simulink model "rx2"  (R2022b)
settings: Solver=FixedStepDiscrete  StartTime=0.0  StopTime=3.3E6  FixedStep=1  RelTol=1e-3  EnableMultiTasking=on
model workspace (MAT data in the model file):
  mwTaskManagerKernelLatency = 0
undefined symbols (not defined in the file or in its folder): Add, jsin, magnitude, rom_pilot_conj_tt, Shift
libraries: hdlsllib x3231, whdlutilities x525, simulink x260, whdlmod x112, whdledac x26, dsphdlmathfun2 x24, commchan3 x1
(part 18 of 59)

== system rx2/process divide/transport_block5/Subsystem1/ctrl_gen ==
  data_in : Inport
  valid_in : Inport  Port=2
  Delay : Delay  DelayLength=1  InitialCondition=0
  Delay1 : Delay  DelayLength=1  InitialCondition=0
  Delay2 : Delay  DelayLength=1  InitialCondition=0
  Detect Fall Nonpositive : hdlsllib/Logic and Bit Operations/Detect Fall Nonpositive  vinit=0  OutDataTypeStr=boolean
  Detect Rise Positive : hdlsllib/Logic and Bit Operations/Detect Rise Positive  vinit=0  OutDataTypeStr=boolean
  Sample Control Bus Creator : whdlutilities/Sample Control Bus Creator
  data_out : Outport
  ctrl_out : Outport  Port=2
  wires:
  Detect Fall Nonpositive/1 -> Sample Control Bus Creator/2
  valid_in/1 -> Delay/1, Detect Fall Nonpositive/1, Delay1/1
  Sample Control Bus Creator/1 -> ctrl_out/1
  Delay/1 -> Sample Control Bus Creator/3
  Delay1/1 -> Detect Rise Positive/1
  data_in/1 -> Delay2/1
  Delay2/1 -> data_out/1
  Detect Rise Positive/1 -> Sample Control Bus Creator/1

== system rx2/process divide/transport_block5/Subsystem10/ctrl_gen ==
  data_in : Inport
  valid_in : Inport  Port=2
  Delay : Delay  DelayLength=1  InitialCondition=0
  Delay1 : Delay  DelayLength=1  InitialCondition=0
  Delay2 : Delay  DelayLength=1  InitialCondition=0
  Detect Fall Nonpositive : hdlsllib/Logic and Bit Operations/Detect Fall Nonpositive  vinit=0  OutDataTypeStr=boolean
  Detect Rise Positive : hdlsllib/Logic and Bit Operations/Detect Rise Positive  vinit=0  OutDataTypeStr=boolean
  Sample Control Bus Creator : whdlutilities/Sample Control Bus Creator
  data_out : Outport
  ctrl_out : Outport  Port=2
  wires:
  Detect Rise Positive/1 -> Sample Control Bus Creator/1
  Delay2/1 -> data_out/1
  data_in/1 -> Delay2/1
  Delay1/1 -> Detect Rise Positive/1
  Delay/1 -> Sample Control Bus Creator/3
  Sample Control Bus Creator/1 -> ctrl_out/1
  valid_in/1 -> Delay1/1, Detect Fall Nonpositive/1, Delay/1
  Detect Fall Nonpositive/1 -> Sample Control Bus Creator/2

== system rx2/process divide/transport_block5/Subsystem11/ctrl_gen ==
  data_in : Inport
  valid_in : Inport  Port=2
  Delay : Delay  DelayLength=1  InitialCondition=0
  Delay1 : Delay  DelayLength=1  InitialCondition=0
  Delay2 : Delay  DelayLength=1  InitialCondition=0
  Detect Fall Nonpositive : hdlsllib/Logic and Bit Operations/Detect Fall Nonpositive  vinit=0  OutDataTypeStr=boolean
  Detect Rise Positive : hdlsllib/Logic and Bit Operations/Detect Rise Positive  vinit=0  OutDataTypeStr=boolean
  Sample Control Bus Creator : whdlutilities/Sample Control Bus Creator
  data_out : Outport
  ctrl_out : Outport  Port=2
  wires:
  Detect Rise Positive/1 -> Sample Control Bus Creator/1
  Delay2/1 -> data_out/1
  data_in/1 -> Delay2/1
  Delay1/1 -> Detect Rise Positive/1
  Delay/1 -> Sample Control Bus Creator/3
  Sample Control Bus Creator/1 -> ctrl_out/1
  valid_in/1 -> Delay1/1, Detect Fall Nonpositive/1, Delay/1
  Detect Fall Nonpositive/1 -> Sample Control Bus Creator/2

== system rx2/process divide/transport_block5/Subsystem12/ctrl_gen ==
  data_in : Inport
  valid_in : Inport  Port=2
  Delay : Delay  DelayLength=1  InitialCondition=0
  Delay1 : Delay  DelayLength=1  InitialCondition=0
  Delay2 : Delay  DelayLength=1  InitialCondition=0
  Detect Fall Nonpositive : hdlsllib/Logic and Bit Operations/Detect Fall Nonpositive  vinit=0  OutDataTypeStr=boolean
  Detect Rise Positive : hdlsllib/Logic and Bit Operations/Detect Rise Positive  vinit=0  OutDataTypeStr=boolean
  Sample Control Bus Creator : whdlutilities/Sample Control Bus Creator
  data_out : Outport
  ctrl_out : Outport  Port=2
  wires:
  Detect Rise Positive/1 -> Sample Control Bus Creator/1
  Delay2/1 -> data_out/1
  data_in/1 -> Delay2/1
  Delay1/1 -> Detect Rise Positive/1
  Delay/1 -> Sample Control Bus Creator/3
  Sample Control Bus Creator/1 -> ctrl_out/1
  valid_in/1 -> Delay1/1, Detect Fall Nonpositive/1, Delay/1
  Detect Fall Nonpositive/1 -> Sample Control Bus Creator/2

== system rx2/process divide/transport_block5/Subsystem13/ctrl_gen ==
  data_in : Inport
  valid_in : Inport  Port=2
  Delay : Delay  DelayLength=1  InitialCondition=0
  Delay1 : Delay  DelayLength=1  InitialCondition=0
  Delay2 : Delay  DelayLength=1  InitialCondition=0
  Detect Fall Nonpositive : hdlsllib/Logic and Bit Operations/Detect Fall Nonpositive  vinit=0  OutDataTypeStr=boolean
  Detect Rise Positive : hdlsllib/Logic and Bit Operations/Detect Rise Positive  vinit=0  OutDataTypeStr=boolean
  Sample Control Bus Creator : whdlutilities/Sample Control Bus Creator
  data_out : Outport
  ctrl_out : Outport  Port=2
  wires:
  Detect Rise Positive/1 -> Sample Control Bus Creator/1
  Delay2/1 -> data_out/1
  data_in/1 -> Delay2/1
  Delay1/1 -> Detect Rise Positive/1
  Delay/1 -> Sample Control Bus Creator/3
  Sample Control Bus Creator/1 -> ctrl_out/1
  valid_in/1 -> Delay1/1, Detect Fall Nonpositive/1, Delay/1
  Detect Fall Nonpositive/1 -> Sample Control Bus Creator/2

== system rx2/process divide/transport_block5/Subsystem14/ctrl_gen ==
  data_in : Inport
  valid_in : Inport  Port=2
  Delay : Delay  DelayLength=1  InitialCondition=0
  Delay1 : Delay  DelayLength=1  InitialCondition=0
  Delay2 : Delay  DelayLength=1  InitialCondition=0
  Detect Fall Nonpositive : hdlsllib/Logic and Bit Operations/Detect Fall Nonpositive  vinit=0  OutDataTypeStr=boolean
  Detect Rise Positive : hdlsllib/Logic and Bit Operations/Detect Rise Positive  vinit=0  OutDataTypeStr=boolean
  Sample Control Bus Creator : whdlutilities/Sample Control Bus Creator
  data_out : Outport
  ctrl_out : Outport  Port=2
  wires:
  Detect Rise Positive/1 -> Sample Control Bus Creator/1
  Delay2/1 -> data_out/1
  data_in/1 -> Delay2/1
  Delay1/1 -> Detect Rise Positive/1
  Delay/1 -> Sample Control Bus Creator/3
  Sample Control Bus Creator/1 -> ctrl_out/1
  valid_in/1 -> Delay1/1, Detect Fall Nonpositive/1, Delay/1
  Detect Fall Nonpositive/1 -> Sample Control Bus Creator/2

== system rx2/process divide/transport_block5/Subsystem2/ctrl_gen ==
  data_in : Inport
  valid_in : Inport  Port=2
  Delay : Delay  DelayLength=1  InitialCondition=0
  Delay1 : Delay  DelayLength=1  InitialCondition=0
  Delay2 : Delay  DelayLength=1  InitialCondition=0
  Detect Fall Nonpositive : hdlsllib/Logic and Bit Operations/Detect Fall Nonpositive  vinit=0  OutDataTypeStr=boolean
  Detect Rise Positive : hdlsllib/Logic and Bit Operations/Detect Rise Positive  vinit=0  OutDataTypeStr=boolean
  Sample Control Bus Creator : whdlutilities/Sample Control Bus Creator
  data_out : Outport
  ctrl_out : Outport  Port=2
  wires:
  Detect Rise Positive/1 -> Sample Control Bus Creator/1
  Delay2/1 -> data_out/1
  data_in/1 -> Delay2/1
  Delay1/1 -> Detect Rise Positive/1
  Delay/1 -> Sample Control Bus Creator/3
  Sample Control Bus Creator/1 -> ctrl_out/1
  valid_in/1 -> Delay1/1, Detect Fall Nonpositive/1, Delay/1
  Detect Fall Nonpositive/1 -> Sample Control Bus Creator/2

== system rx2/process divide/transport_block5/Subsystem3/ctrl_gen ==
  data_in : Inport
  valid_in : Inport  Port=2
  Delay : Delay  DelayLength=1  InitialCondition=0
  Delay1 : Delay  DelayLength=1  InitialCondition=0
  Delay2 : Delay  DelayLength=1  InitialCondition=0
  Detect Fall Nonpositive : hdlsllib/Logic and Bit Operations/Detect Fall Nonpositive  vinit=0  OutDataTypeStr=boolean
  Detect Rise Positive : hdlsllib/Logic and Bit Operations/Detect Rise Positive  vinit=0  OutDataTypeStr=boolean
  Sample Control Bus Creator : whdlutilities/Sample Control Bus Creator
  data_out : Outport
  ctrl_out : Outport  Port=2
  wires:
  Detect Fall Nonpositive/1 -> Sample Control Bus Creator/2
  valid_in/1 -> Delay/1, Detect Fall Nonpositive/1, Delay1/1
  Sample Control Bus Creator/1 -> ctrl_out/1
  Delay/1 -> Sample Control Bus Creator/3
  Delay1/1 -> Detect Rise Positive/1
  data_in/1 -> Delay2/1
  Delay2/1 -> data_out/1
  Detect Rise Positive/1 -> Sample Control Bus Creator/1

== system rx2/process divide/transport_block5/Subsystem4/ctrl_gen ==
  data_in : Inport
  valid_in : Inport  Port=2
  Delay : Delay  DelayLength=1  InitialCondition=0
  Delay1 : Delay  DelayLength=1  InitialCondition=0
  Delay2 : Delay  DelayLength=1  InitialCondition=0
  Detect Fall Nonpositive : hdlsllib/Logic and Bit Operations/Detect Fall Nonpositive  vinit=0  OutDataTypeStr=boolean
  Detect Rise Positive : hdlsllib/Logic and Bit Operations/Detect Rise Positive  vinit=0  OutDataTypeStr=boolean
  Sample Control Bus Creator : whdlutilities/Sample Control Bus Creator
  data_out : Outport
  ctrl_out : Outport  Port=2
  wires:
  Detect Rise Positive/1 -> Sample Control Bus Creator/1
  Delay2/1 -> data_out/1
  data_in/1 -> Delay2/1
  Delay1/1 -> Detect Rise Positive/1
  Delay/1 -> Sample Control Bus Creator/3
  Sample Control Bus Creator/1 -> ctrl_out/1
  valid_in/1 -> Delay1/1, Detect Fall Nonpositive/1, Delay/1
  Detect Fall Nonpositive/1 -> Sample Control Bus Creator/2

== system rx2/process divide/transport_block5/Subsystem5/ctrl_gen ==
  data_in : Inport
  valid_in : Inport  Port=2
  Delay : Delay  DelayLength=1  InitialCondition=0
  Delay1 : Delay  DelayLength=1  InitialCondition=0
  Delay2 : Delay  DelayLength=1  InitialCondition=0
  Detect Fall Nonpositive : hdlsllib/Logic and Bit Operations/Detect Fall Nonpositive  vinit=0  OutDataTypeStr=boolean
  Detect Rise Positive : hdlsllib/Logic and Bit Operations/Detect Rise Positive  vinit=0  OutDataTypeStr=boolean
  Sample Control Bus Creator : whdlutilities/Sample Control Bus Creator
  data_out : Outport
  ctrl_out : Outport  Port=2
  wires:
  Detect Rise Positive/1 -> Sample Control Bus Creator/1
  Delay2/1 -> data_out/1
  data_in/1 -> Delay2/1
  Delay1/1 -> Detect Rise Positive/1
  Delay/1 -> Sample Control Bus Creator/3
  Sample Control Bus Creator/1 -> ctrl_out/1
  valid_in/1 -> Delay1/1, Detect Fall Nonpositive/1, Delay/1
  Detect Fall Nonpositive/1 -> Sample Control Bus Creator/2

== system rx2/process divide/transport_block5/Subsystem6/ctrl_gen ==
  data_in : Inport
  valid_in : Inport  Port=2
  Delay : Delay  DelayLength=1  InitialCondition=0
  Delay1 : Delay  DelayLength=1  InitialCondition=0
  Delay2 : Delay  DelayLength=1  InitialCondition=0
  Detect Fall Nonpositive : hdlsllib/Logic and Bit Operations/Detect Fall Nonpositive  vinit=0  OutDataTypeStr=boolean
  Detect Rise Positive : hdlsllib/Logic and Bit Operations/Detect Rise Positive  vinit=0  OutDataTypeStr=boolean
  Sample Control Bus Creator : whdlutilities/Sample Control Bus Creator
  data_out : Outport
  ctrl_out : Outport  Port=2
  wires:
  Detect Rise Positive/1 -> Sample Control Bus Creator/1
  Delay2/1 -> data_out/1
  data_in/1 -> Delay2/1
  Delay1/1 -> Detect Rise Positive/1
  Delay/1 -> Sample Control Bus Creator/3
  Sample Control Bus Creator/1 -> ctrl_out/1
  valid_in/1 -> Delay1/1, Detect Fall Nonpositive/1, Delay/1
  Detect Fall Nonpositive/1 -> Sample Control Bus Creator/2

== system rx2/process divide/transport_block5/Subsystem7/ctrl_gen ==
  data_in : Inport
  valid_in : Inport  Port=2
  Delay : Delay  DelayLength=1  InitialCondition=0
  Delay1 : Delay  DelayLength=1  InitialCondition=0
  Delay2 : Delay  DelayLength=1  InitialCondition=0
  Detect Fall Nonpositive : hdlsllib/Logic and Bit Operations/Detect Fall Nonpositive  vinit=0  OutDataTypeStr=boolean
  Detect Rise Positive : hdlsllib/Logic and Bit Operations/Detect Rise Positive  vinit=0  OutDataTypeStr=boolean
  Sample Control Bus Creator : whdlutilities/Sample Control Bus Creator
  data_out : Outport
  ctrl_out : Outport  Port=2
  wires:
  Detect Rise Positive/1 -> Sample Control Bus Creator/1
  Delay2/1 -> data_out/1
  data_in/1 -> Delay2/1
  Delay1/1 -> Detect Rise Positive/1
  Delay/1 -> Sample Control Bus Creator/3
  Sample Control Bus Creator/1 -> ctrl_out/1
  valid_in/1 -> Delay1/1, Detect Fall Nonpositive/1, Delay/1
  Detect Fall Nonpositive/1 -> Sample Control Bus Creator/2

== system rx2/process divide/transport_block5/Subsystem8/ctrl_gen ==
  data_in : Inport
  valid_in : Inport  Port=2
  Delay : Delay  DelayLength=1  InitialCondition=0
  Delay1 : Delay  DelayLength=1  InitialCondition=0
  Delay2 : Delay  DelayLength=1  InitialCondition=0
  Detect Fall Nonpositive : hdlsllib/Logic and Bit Operations/Detect Fall Nonpositive  vinit=0  OutDataTypeStr=boolean
  Detect Rise Positive : hdlsllib/Logic and Bit Operations/Detect Rise Positive  vinit=0  OutDataTypeStr=boolean
  Sample Control Bus Creator : whdlutilities/Sample Control Bus Creator
  data_out : Outport
  ctrl_out : Outport  Port=2
  wires:
  Detect Rise Positive/1 -> Sample Control Bus Creator/1
  Delay2/1 -> data_out/1
  data_in/1 -> Delay2/1
  Delay1/1 -> Detect Rise Positive/1
  Delay/1 -> Sample Control Bus Creator/3
  Sample Control Bus Creator/1 -> ctrl_out/1
  valid_in/1 -> Delay1/1, Detect Fall Nonpositive/1, Delay/1
  Detect Fall Nonpositive/1 -> Sample Control Bus Creator/2

== system rx2/process divide/transport_block5/Subsystem9/ctrl_gen ==
  data_in : Inport
  valid_in : Inport  Port=2
  Delay : Delay  DelayLength=1  InitialCondition=0
  Delay1 : Delay  DelayLength=1  InitialCondition=0
  Delay2 : Delay  DelayLength=1  InitialCondition=0
  Detect Fall Nonpositive : hdlsllib/Logic and Bit Operations/Detect Fall Nonpositive  vinit=0  OutDataTypeStr=boolean
  Detect Rise Positive : hdlsllib/Logic and Bit Operations/Detect Rise Positive  vinit=0  OutDataTypeStr=boolean
  Sample Control Bus Creator : whdlutilities/Sample Control Bus Creator
  data_out : Outport
  ctrl_out : Outport  Port=2
  wires:
  Detect Rise Positive/1 -> Sample Control Bus Creator/1
  Delay2/1 -> data_out/1
  data_in/1 -> Delay2/1
  Delay1/1 -> Detect Rise Positive/1
  Delay/1 -> Sample Control Bus Creator/3
  Sample Control Bus Creator/1 -> ctrl_out/1
  valid_in/1 -> Delay1/1, Detect Fall Nonpositive/1, Delay/1
  Detect Fall Nonpositive/1 -> Sample Control Bus Creator/2

== system rx2/process divide/transport_block6/Subsystem1/ctrl_gen ==
  data_in : Inport
  valid_in : Inport  Port=2
  Delay : Delay  DelayLength=1  InitialCondition=0
  Delay1 : Delay  DelayLength=1  InitialCondition=0
  Delay2 : Delay  DelayLength=1  InitialCondition=0
  Detect Fall Nonpositive : hdlsllib/Logic and Bit Operations/Detect Fall Nonpositive  vinit=0  OutDataTypeStr=boolean
  Detect Rise Positive : hdlsllib/Logic and Bit Operations/Detect Rise Positive  vinit=0  OutDataTypeStr=boolean
  Sample Control Bus Creator : whdlutilities/Sample Control Bus Creator
  data_out : Outport
  ctrl_out : Outport  Port=2
  wires:
  Detect Rise Positive/1 -> Sample Control Bus Creator/1
  Delay2/1 -> data_out/1
  data_in/1 -> Delay2/1
  Delay1/1 -> Detect Rise Positive/1
  Delay/1 -> Sample Control Bus Creator/3
  Sample Control Bus Creator/1 -> ctrl_out/1
  valid_in/1 -> Delay1/1, Detect Fall Nonpositive/1, Delay/1
  Detect Fall Nonpositive/1 -> Sample Control Bus Creator/2

== system rx2/process divide/transport_block6/Subsystem10/ctrl_gen ==
  data_in : Inport
  valid_in : Inport  Port=2
  Delay : Delay  DelayLength=1  InitialCondition=0
  Delay1 : Delay  DelayLength=1  InitialCondition=0
  Delay2 : Delay  DelayLength=1  InitialCondition=0
  Detect Fall Nonpositive : hdlsllib/Logic and Bit Operations/Detect Fall Nonpositive  vinit=0  OutDataTypeStr=boolean
  Detect Rise Positive : hdlsllib/Logic and Bit Operations/Detect Rise Positive  vinit=0  OutDataTypeStr=boolean
  Sample Control Bus Creator : whdlutilities/Sample Control Bus Creator
  data_out : Outport
  ctrl_out : Outport  Port=2
  wires:
  Detect Fall Nonpositive/1 -> Sample Control Bus Creator/2
  valid_in/1 -> Delay/1, Detect Fall Nonpositive/1, Delay1/1
  Sample Control Bus Creator/1 -> ctrl_out/1
  Delay/1 -> Sample Control Bus Creator/3
  Delay1/1 -> Detect Rise Positive/1
  data_in/1 -> Delay2/1
  Delay2/1 -> data_out/1
  Detect Rise Positive/1 -> Sample Control Bus Creator/1

== system rx2/process divide/transport_block6/Subsystem11/ctrl_gen ==
  data_in : Inport
  valid_in : Inport  Port=2
  Delay : Delay  DelayLength=1  InitialCondition=0
  Delay1 : Delay  DelayLength=1  InitialCondition=0
  Delay2 : Delay  DelayLength=1  InitialCondition=0
  Detect Fall Nonpositive : hdlsllib/Logic and Bit Operations/Detect Fall Nonpositive  vinit=0  OutDataTypeStr=boolean
  Detect Rise Positive : hdlsllib/Logic and Bit Operations/Detect Rise Positive  vinit=0  OutDataTypeStr=boolean
  Sample Control Bus Creator : whdlutilities/Sample Control Bus Creator
  data_out : Outport
  ctrl_out : Outport  Port=2
  wires:
  Detect Fall Nonpositive/1 -> Sample Control Bus Creator/2
  valid_in/1 -> Delay/1, Detect Fall Nonpositive/1, Delay1/1
  Sample Control Bus Creator/1 -> ctrl_out/1
  Delay/1 -> Sample Control Bus Creator/3
  Delay1/1 -> Detect Rise Positive/1
  data_in/1 -> Delay2/1
  Delay2/1 -> data_out/1
  Detect Rise Positive/1 -> Sample Control Bus Creator/1

== system rx2/process divide/transport_block6/Subsystem12/ctrl_gen ==
  data_in : Inport
  valid_in : Inport  Port=2
  Delay : Delay  DelayLength=1  InitialCondition=0
  Delay1 : Delay  DelayLength=1  InitialCondition=0
  Delay2 : Delay  DelayLength=1  InitialCondition=0
  Detect Fall Nonpositive : hdlsllib/Logic and Bit Operations/Detect Fall Nonpositive  vinit=0  OutDataTypeStr=boolean
  Detect Rise Positive : hdlsllib/Logic and Bit Operations/Detect Rise Positive  vinit=0  OutDataTypeStr=boolean
  Sample Control Bus Creator : whdlutilities/Sample Control Bus Creator
  data_out : Outport
  ctrl_out : Outport  Port=2
  wires:
  Detect Fall Nonpositive/1 -> Sample Control Bus Creator/2
  valid_in/1 -> Delay/1, Detect Fall Nonpositive/1, Delay1/1
  Sample Control Bus Creator/1 -> ctrl_out/1
  Delay/1 -> Sample Control Bus Creator/3
  Delay1/1 -> Detect Rise Positive/1
  data_in/1 -> Delay2/1
  Delay2/1 -> data_out/1
  Detect Rise Positive/1 -> Sample Control Bus Creator/1

== system rx2/process divide/transport_block6/Subsystem13/ctrl_gen ==
  data_in : Inport
  valid_in : Inport  Port=2
  Delay : Delay  DelayLength=1  InitialCondition=0
  Delay1 : Delay  DelayLength=1  InitialCondition=0
  Delay2 : Delay  DelayLength=1  InitialCondition=0
  Detect Fall Nonpositive : hdlsllib/Logic and Bit Operations/Detect Fall Nonpositive  vinit=0  OutDataTypeStr=boolean
  Detect Rise Positive : hdlsllib/Logic and Bit Operations/Detect Rise Positive  vinit=0  OutDataTypeStr=boolean
  Sample Control Bus Creator : whdlutilities/Sample Control Bus Creator
  data_out : Outport
  ctrl_out : Outport  Port=2
  wires:
  Detect Fall Nonpositive/1 -> Sample Control Bus Creator/2
  valid_in/1 -> Delay/1, Detect Fall Nonpositive/1, Delay1/1
  Sample Control Bus Creator/1 -> ctrl_out/1
  Delay/1 -> Sample Control Bus Creator/3
  Delay1/1 -> Detect Rise Positive/1
  data_in/1 -> Delay2/1
  Delay2/1 -> data_out/1
  Detect Rise Positive/1 -> Sample Control Bus Creator/1

== system rx2/process divide/transport_block6/Subsystem14/ctrl_gen ==
  data_in : Inport
  valid_in : Inport  Port=2
  Delay : Delay  DelayLength=1  InitialCondition=0
  Delay1 : Delay  DelayLength=1  InitialCondition=0
  Delay2 : Delay  DelayLength=1  InitialCondition=0
  Detect Fall Nonpositive : hdlsllib/Logic and Bit Operations/Detect Fall Nonpositive  vinit=0  OutDataTypeStr=boolean
  Detect Rise Positive : hdlsllib/Logic and Bit Operations/Detect Rise Positive  vinit=0  OutDataTypeStr=boolean
  Sample Control Bus Creator : whdlutilities/Sample Control Bus Creator
  data_out : Outport
  ctrl_out : Outport  Port=2
  wires:
  Detect Fall Nonpositive/1 -> Sample Control Bus Creator/2
  valid_in/1 -> Delay/1, Detect Fall Nonpositive/1, Delay1/1
  Sample Control Bus Creator/1 -> ctrl_out/1
  Delay/1 -> Sample Control Bus Creator/3
  Delay1/1 -> Detect Rise Positive/1
  data_in/1 -> Delay2/1
  Delay2/1 -> data_out/1
  Detect Rise Positive/1 -> Sample Control Bus Creator/1

== system rx2/process divide/transport_block6/Subsystem2/ctrl_gen ==
  data_in : Inport
  valid_in : Inport  Port=2
  Delay : Delay  DelayLength=1  InitialCondition=0
  Delay1 : Delay  DelayLength=1  InitialCondition=0
  Delay2 : Delay  DelayLength=1  InitialCondition=0
  Detect Fall Nonpositive : hdlsllib/Logic and Bit Operations/Detect Fall Nonpositive  vinit=0  OutDataTypeStr=boolean
  Detect Rise Positive : hdlsllib/Logic and Bit Operations/Detect Rise Positive  vinit=0  OutDataTypeStr=boolean
  Sample Control Bus Creator : whdlutilities/Sample Control Bus Creator
  data_out : Outport
  ctrl_out : Outport  Port=2
  wires:
  Detect Fall Nonpositive/1 -> Sample Control Bus Creator/2
  valid_in/1 -> Delay/1, Detect Fall Nonpositive/1, Delay1/1
  Sample Control Bus Creator/1 -> ctrl_out/1
  Delay/1 -> Sample Control Bus Creator/3
  Delay1/1 -> Detect Rise Positive/1
  data_in/1 -> Delay2/1
  Delay2/1 -> data_out/1
  Detect Rise Positive/1 -> Sample Control Bus Creator/1

== system rx2/process divide/transport_block6/Subsystem3/ctrl_gen ==
  data_in : Inport
  valid_in : Inport  Port=2
  Delay : Delay  DelayLength=1  InitialCondition=0
  Delay1 : Delay  DelayLength=1  InitialCondition=0
  Delay2 : Delay  DelayLength=1  InitialCondition=0
  Detect Fall Nonpositive : hdlsllib/Logic and Bit Operations/Detect Fall Nonpositive  vinit=0  OutDataTypeStr=boolean
  Detect Rise Positive : hdlsllib/Logic and Bit Operations/Detect Rise Positive  vinit=0  OutDataTypeStr=boolean
  Sample Control Bus Creator : whdlutilities/Sample Control Bus Creator
  data_out : Outport
  ctrl_out : Outport  Port=2
  wires:
  Detect Rise Positive/1 -> Sample Control Bus Creator/1
  Delay2/1 -> data_out/1
  data_in/1 -> Delay2/1
  Delay1/1 -> Detect Rise Positive/1
  Delay/1 -> Sample Control Bus Creator/3
  Sample Control Bus Creator/1 -> ctrl_out/1
  valid_in/1 -> Delay1/1, Detect Fall Nonpositive/1, Delay/1
  Detect Fall Nonpositive/1 -> Sample Control Bus Creator/2

== system rx2/process divide/transport_block6/Subsystem4/ctrl_gen ==
  data_in : Inport
  valid_in : Inport  Port=2
  Delay : Delay  DelayLength=1  InitialCondition=0
  Delay1 : Delay  DelayLength=1  InitialCondition=0
  Delay2 : Delay  DelayLength=1  InitialCondition=0
  Detect Fall Nonpositive : hdlsllib/Logic and Bit Operations/Detect Fall Nonpositive  vinit=0  OutDataTypeStr=boolean
  Detect Rise Positive : hdlsllib/Logic and Bit Operations/Detect Rise Positive  vinit=0  OutDataTypeStr=boolean
  Sample Control Bus Creator : whdlutilities/Sample Control Bus Creator
  data_out : Outport
  ctrl_out : Outport  Port=2
  wires:
  Detect Fall Nonpositive/1 -> Sample Control Bus Creator/2
  valid_in/1 -> Delay/1, Detect Fall Nonpositive/1, Delay1/1
  Sample Control Bus Creator/1 -> ctrl_out/1
  Delay/1 -> Sample Control Bus Creator/3
  Delay1/1 -> Detect Rise Positive/1
  data_in/1 -> Delay2/1
  Delay2/1 -> data_out/1
  Detect Rise Positive/1 -> Sample Control Bus Creator/1

== system rx2/process divide/transport_block6/Subsystem5/ctrl_gen ==
  data_in : Inport
  valid_in : Inport  Port=2
  Delay : Delay  DelayLength=1  InitialCondition=0
  Delay1 : Delay  DelayLength=1  InitialCondition=0
  Delay2 : Delay  DelayLength=1  InitialCondition=0
  Detect Fall Nonpositive : hdlsllib/Logic and Bit Operations/Detect Fall Nonpositive  vinit=0  OutDataTypeStr=boolean
  Detect Rise Positive : hdlsllib/Logic and Bit Operations/Detect Rise Positive  vinit=0  OutDataTypeStr=boolean
  Sample Control Bus Creator : whdlutilities/Sample Control Bus Creator
  data_out : Outport
  ctrl_out : Outport  Port=2
  wires:
  Detect Fall Nonpositive/1 -> Sample Control Bus Creator/2
  valid_in/1 -> Delay/1, Detect Fall Nonpositive/1, Delay1/1
  Sample Control Bus Creator/1 -> ctrl_out/1
  Delay/1 -> Sample Control Bus Creator/3
  Delay1/1 -> Detect Rise Positive/1
  data_in/1 -> Delay2/1
  Delay2/1 -> data_out/1
  Detect Rise Positive/1 -> Sample Control Bus Creator/1

== system rx2/process divide/transport_block6/Subsystem6/ctrl_gen ==
  data_in : Inport
  valid_in : Inport  Port=2
  Delay : Delay  DelayLength=1  InitialCondition=0
  Delay1 : Delay  DelayLength=1  InitialCondition=0
  Delay2 : Delay  DelayLength=1  InitialCondition=0
  Detect Fall Nonpositive : hdlsllib/Logic and Bit Operations/Detect Fall Nonpositive  vinit=0  OutDataTypeStr=boolean
  Detect Rise Positive : hdlsllib/Logic and Bit Operations/Detect Rise Positive  vinit=0  OutDataTypeStr=boolean
  Sample Control Bus Creator : whdlutilities/Sample Control Bus Creator
  data_out : Outport
  ctrl_out : Outport  Port=2
  wires:
  Detect Fall Nonpositive/1 -> Sample Control Bus Creator/2
  valid_in/1 -> Delay/1, Detect Fall Nonpositive/1, Delay1/1
  Sample Control Bus Creator/1 -> ctrl_out/1
  Delay/1 -> Sample Control Bus Creator/3
  Delay1/1 -> Detect Rise Positive/1
  data_in/1 -> Delay2/1
  Delay2/1 -> data_out/1
  Detect Rise Positive/1 -> Sample Control Bus Creator/1

== system rx2/process divide/transport_block6/Subsystem7/ctrl_gen ==
  data_in : Inport
  valid_in : Inport  Port=2
  Delay : Delay  DelayLength=1  InitialCondition=0
  Delay1 : Delay  DelayLength=1  InitialCondition=0
  Delay2 : Delay  DelayLength=1  InitialCondition=0
  Detect Fall Nonpositive : hdlsllib/Logic and Bit Operations/Detect Fall Nonpositive  vinit=0  OutDataTypeStr=boolean
  Detect Rise Positive : hdlsllib/Logic and Bit Operations/Detect Rise Positive  vinit=0  OutDataTypeStr=boolean
  Sample Control Bus Creator : whdlutilities/Sample Control Bus Creator
  data_out : Outport
  ctrl_out : Outport  Port=2
  wires:
  Detect Fall Nonpositive/1 -> Sample Control Bus Creator/2
  valid_in/1 -> Delay/1, Detect Fall Nonpositive/1, Delay1/1
  Sample Control Bus Creator/1 -> ctrl_out/1
  Delay/1 -> Sample Control Bus Creator/3
  Delay1/1 -> Detect Rise Positive/1
  data_in/1 -> Delay2/1
  Delay2/1 -> data_out/1
  Detect Rise Positive/1 -> Sample Control Bus Creator/1

== system rx2/process divide/transport_block6/Subsystem8/ctrl_gen ==
  data_in : Inport
  valid_in : Inport  Port=2
  Delay : Delay  DelayLength=1  InitialCondition=0
  Delay1 : Delay  DelayLength=1  InitialCondition=0
  Delay2 : Delay  DelayLength=1  InitialCondition=0
  Detect Fall Nonpositive : hdlsllib/Logic and Bit Operations/Detect Fall Nonpositive  vinit=0  OutDataTypeStr=boolean
  Detect Rise Positive : hdlsllib/Logic and Bit Operations/Detect Rise Positive  vinit=0  OutDataTypeStr=boolean
  Sample Control Bus Creator : whdlutilities/Sample Control Bus Creator
  data_out : Outport
  ctrl_out : Outport  Port=2
  wires:
  Detect Fall Nonpositive/1 -> Sample Control Bus Creator/2
  valid_in/1 -> Delay/1, Detect Fall Nonpositive/1, Delay1/1
  Sample Control Bus Creator/1 -> ctrl_out/1
  Delay/1 -> Sample Control Bus Creator/3
  Delay1/1 -> Detect Rise Positive/1
  data_in/1 -> Delay2/1
  Delay2/1 -> data_out/1
  Detect Rise Positive/1 -> Sample Control Bus Creator/1

== system rx2/process divide/transport_block6/Subsystem9/ctrl_gen ==
  data_in : Inport
  valid_in : Inport  Port=2
  Delay : Delay  DelayLength=1  InitialCondition=0
  Delay1 : Delay  DelayLength=1  InitialCondition=0
  Delay2 : Delay  DelayLength=1  InitialCondition=0
  Detect Fall Nonpositive : hdlsllib/Logic and Bit Operations/Detect Fall Nonpositive  vinit=0  OutDataTypeStr=boolean
  Detect Rise Positive : hdlsllib/Logic and Bit Operations/Detect Rise Positive  vinit=0  OutDataTypeStr=boolean
  Sample Control Bus Creator : whdlutilities/Sample Control Bus Creator
  data_out : Outport
  ctrl_out : Outport  Port=2
  wires:
  Detect Fall Nonpositive/1 -> Sample Control Bus Creator/2
  valid_in/1 -> Delay/1, Detect Fall Nonpositive/1, Delay1/1
  Sample Control Bus Creator/1 -> ctrl_out/1
  Delay/1 -> Sample Control Bus Creator/3
  Delay1/1 -> Detect Rise Positive/1
  data_in/1 -> Delay2/1
  Delay2/1 -> data_out/1
  Detect Rise Positive/1 -> Sample Control Bus Creator/1

== system rx2/process divide/transport_block7/Subsystem1/ctrl_gen ==
  data_in : Inport
  valid_in : Inport  Port=2
  Delay : Delay  DelayLength=1  InitialCondition=0
  Delay1 : Delay  DelayLength=1  InitialCondition=0
  Delay2 : Delay  DelayLength=1  InitialCondition=0
  Detect Fall Nonpositive : hdlsllib/Logic and Bit Operations/Detect Fall Nonpositive  vinit=0  OutDataTypeStr=boolean
  Detect Rise Positive : hdlsllib/Logic and Bit Operations/Detect Rise Positive  vinit=0  OutDataTypeStr=boolean
  Sample Control Bus Creator : whdlutilities/Sample Control Bus Creator
  data_out : Outport
  ctrl_out : Outport  Port=2
  wires:
  Detect Fall Nonpositive/1 -> Sample Control Bus Creator/2
  valid_in/1 -> Delay/1, Detect Fall Nonpositive/1, Delay1/1
  Sample Control Bus Creator/1 -> ctrl_out/1
  Delay/1 -> Sample Control Bus Creator/3
  Delay1/1 -> Detect Rise Positive/1
  data_in/1 -> Delay2/1
  Delay2/1 -> data_out/1
  Detect Rise Positive/1 -> Sample Control Bus Creator/1

== system rx2/process divide/transport_block7/Subsystem10/ctrl_gen ==
  data_in : Inport
  valid_in : Inport  Port=2
  Delay : Delay  DelayLength=1  InitialCondition=0
  Delay1 : Delay  DelayLength=1  InitialCondition=0
  Delay2 : Delay  DelayLength=1  InitialCondition=0
  Detect Fall Nonpositive : hdlsllib/Logic and Bit Operations/Detect Fall Nonpositive  vinit=0  OutDataTypeStr=boolean
  Detect Rise Positive : hdlsllib/Logic and Bit Operations/Detect Rise Positive  vinit=0  OutDataTypeStr=boolean
  Sample Control Bus Creator : whdlutilities/Sample Control Bus Creator
  data_out : Outport
  ctrl_out : Outport  Port=2
  wires:
  Detect Rise Positive/1 -> Sample Control Bus Creator/1
  Delay2/1 -> data_out/1
  data_in/1 -> Delay2/1
  Delay1/1 -> Detect Rise Positive/1
  Delay/1 -> Sample Control Bus Creator/3
  Sample Control Bus Creator/1 -> ctrl_out/1
  valid_in/1 -> Delay1/1, Detect Fall Nonpositive/1, Delay/1
  Detect Fall Nonpositive/1 -> Sample Control Bus Creator/2

== system rx2/process divide/transport_block7/Subsystem11/ctrl_gen ==
  data_in : Inport
  valid_in : Inport  Port=2
  Delay : Delay  DelayLength=1  InitialCondition=0
  Delay1 : Delay  DelayLength=1  InitialCondition=0
  Delay2 : Delay  DelayLength=1  InitialCondition=0
  Detect Fall Nonpositive : hdlsllib/Logic and Bit Operations/Detect Fall Nonpositive  vinit=0  OutDataTypeStr=boolean
  Detect Rise Positive : hdlsllib/Logic and Bit Operations/Detect Rise Positive  vinit=0  OutDataTypeStr=boolean
  Sample Control Bus Creator : whdlutilities/Sample Control Bus Creator
  data_out : Outport
  ctrl_out : Outport  Port=2
  wires:
  Detect Rise Positive/1 -> Sample Control Bus Creator/1
  Delay2/1 -> data_out/1
  data_in/1 -> Delay2/1
  Delay1/1 -> Detect Rise Positive/1
  Delay/1 -> Sample Control Bus Creator/3
  Sample Control Bus Creator/1 -> ctrl_out/1
  valid_in/1 -> Delay1/1, Detect Fall Nonpositive/1, Delay/1
  Detect Fall Nonpositive/1 -> Sample Control Bus Creator/2

== system rx2/process divide/transport_block7/Subsystem12/ctrl_gen ==
  data_in : Inport
  valid_in : Inport  Port=2
  Delay : Delay  DelayLength=1  InitialCondition=0
  Delay1 : Delay  DelayLength=1  InitialCondition=0
  Delay2 : Delay  DelayLength=1  InitialCondition=0
  Detect Fall Nonpositive : hdlsllib/Logic and Bit Operations/Detect Fall Nonpositive  vinit=0  OutDataTypeStr=boolean
  Detect Rise Positive : hdlsllib/Logic and Bit Operations/Detect Rise Positive  vinit=0  OutDataTypeStr=boolean
  Sample Control Bus Creator : whdlutilities/Sample Control Bus Creator
  data_out : Outport
  ctrl_out : Outport  Port=2
  wires:
  Detect Rise Positive/1 -> Sample Control Bus Creator/1
  Delay2/1 -> data_out/1
  data_in/1 -> Delay2/1
  Delay1/1 -> Detect Rise Positive/1
  Delay/1 -> Sample Control Bus Creator/3
  Sample Control Bus Creator/1 -> ctrl_out/1
  valid_in/1 -> Delay1/1, Detect Fall Nonpositive/1, Delay/1
  Detect Fall Nonpositive/1 -> Sample Control Bus Creator/2

== system rx2/process divide/transport_block7/Subsystem13/ctrl_gen ==
  data_in : Inport
  valid_in : Inport  Port=2
  Delay : Delay  DelayLength=1  InitialCondition=0
  Delay1 : Delay  DelayLength=1  InitialCondition=0
  Delay2 : Delay  DelayLength=1  InitialCondition=0
  Detect Fall Nonpositive : hdlsllib/Logic and Bit Operations/Detect Fall Nonpositive  vinit=0  OutDataTypeStr=boolean
  Detect Rise Positive : hdlsllib/Logic and Bit Operations/Detect Rise Positive  vinit=0  OutDataTypeStr=boolean
  Sample Control Bus Creator : whdlutilities/Sample Control Bus Creator
  data_out : Outport
  ctrl_out : Outport  Port=2
  wires:
  Detect Rise Positive/1 -> Sample Control Bus Creator/1
  Delay2/1 -> data_out/1
  data_in/1 -> Delay2/1
  Delay1/1 -> Detect Rise Positive/1
  Delay/1 -> Sample Control Bus Creator/3
  Sample Control Bus Creator/1 -> ctrl_out/1
  valid_in/1 -> Delay1/1, Detect Fall Nonpositive/1, Delay/1
  Detect Fall Nonpositive/1 -> Sample Control Bus Creator/2

== system rx2/process divide/transport_block7/Subsystem14/ctrl_gen ==
  data_in : Inport
  valid_in : Inport  Port=2
  Delay : Delay  DelayLength=1  InitialCondition=0
  Delay1 : Delay  DelayLength=1  InitialCondition=0
  Delay2 : Delay  DelayLength=1  InitialCondition=0
  Detect Fall Nonpositive : hdlsllib/Logic and Bit Operations/Detect Fall Nonpositive  vinit=0  OutDataTypeStr=boolean
  Detect Rise Positive : hdlsllib/Logic and Bit Operations/Detect Rise Positive  vinit=0  OutDataTypeStr=boolean
  Sample Control Bus Creator : whdlutilities/Sample Control Bus Creator
  data_out : Outport
  ctrl_out : Outport  Port=2
  wires:
  Detect Rise Positive/1 -> Sample Control Bus Creator/1
  Delay2/1 -> data_out/1
  data_in/1 -> Delay2/1
  Delay1/1 -> Detect Rise Positive/1
  Delay/1 -> Sample Control Bus Creator/3
  Sample Control Bus Creator/1 -> ctrl_out/1
  valid_in/1 -> Delay1/1, Detect Fall Nonpositive/1, Delay/1
  Detect Fall Nonpositive/1 -> Sample Control Bus Creator/2

== system rx2/process divide/transport_block7/Subsystem2/ctrl_gen ==
  data_in : Inport
  valid_in : Inport  Port=2
  Delay : Delay  DelayLength=1  InitialCondition=0
  Delay1 : Delay  DelayLength=1  InitialCondition=0
  Delay2 : Delay  DelayLength=1  InitialCondition=0
  Detect Fall Nonpositive : hdlsllib/Logic and Bit Operations/Detect Fall Nonpositive  vinit=0  OutDataTypeStr=boolean
  Detect Rise Positive : hdlsllib/Logic and Bit Operations/Detect Rise Positive  vinit=0  OutDataTypeStr=boolean
  Sample Control Bus Creator : whdlutilities/Sample Control Bus Creator
  data_out : Outport
  ctrl_out : Outport  Port=2
  wires:
  Detect Rise Positive/1 -> Sample Control Bus Creator/1
  Delay2/1 -> data_out/1
  data_in/1 -> Delay2/1
  Delay1/1 -> Detect Rise Positive/1
  Delay/1 -> Sample Control Bus Creator/3
  Sample Control Bus Creator/1 -> ctrl_out/1
  valid_in/1 -> Delay1/1, Detect Fall Nonpositive/1, Delay/1
  Detect Fall Nonpositive/1 -> Sample Control Bus Creator/2

== system rx2/process divide/transport_block7/Subsystem3/ctrl_gen ==
  data_in : Inport
  valid_in : Inport  Port=2
  Delay : Delay  DelayLength=1  InitialCondition=0
  Delay1 : Delay  DelayLength=1  InitialCondition=0
  Delay2 : Delay  DelayLength=1  InitialCondition=0
  Detect Fall Nonpositive : hdlsllib/Logic and Bit Operations/Detect Fall Nonpositive  vinit=0  OutDataTypeStr=boolean
  Detect Rise Positive : hdlsllib/Logic and Bit Operations/Detect Rise Positive  vinit=0  OutDataTypeStr=boolean
  Sample Control Bus Creator : whdlutilities/Sample Control Bus Creator
  data_out : Outport
  ctrl_out : Outport  Port=2
  wires:
  Detect Fall Nonpositive/1 -> Sample Control Bus Creator/2
  valid_in/1 -> Delay/1, Detect Fall Nonpositive/1, Delay1/1
  Sample Control Bus Creator/1 -> ctrl_out/1
  Delay/1 -> Sample Control Bus Creator/3
  Delay1/1 -> Detect Rise Positive/1
  data_in/1 -> Delay2/1
  Delay2/1 -> data_out/1
  Detect Rise Positive/1 -> Sample Control Bus Creator/1

== system rx2/process divide/transport_block7/Subsystem4/ctrl_gen ==
  data_in : Inport
  valid_in : Inport  Port=2
  Delay : Delay  DelayLength=1  InitialCondition=0
  Delay1 : Delay  DelayLength=1  InitialCondition=0
  Delay2 : Delay  DelayLength=1  InitialCondition=0
  Detect Fall Nonpositive : hdlsllib/Logic and Bit Operations/Detect Fall Nonpositive  vinit=0  OutDataTypeStr=boolean
  Detect Rise Positive : hdlsllib/Logic and Bit Operations/Detect Rise Positive  vinit=0  OutDataTypeStr=boolean
  Sample Control Bus Creator : whdlutilities/Sample Control Bus Creator
  data_out : Outport
  ctrl_out : Outport  Port=2
  wires:
  Detect Rise Positive/1 -> Sample Control Bus Creator/1
  Delay2/1 -> data_out/1
  data_in/1 -> Delay2/1
  Delay1/1 -> Detect Rise Positive/1
  Delay/1 -> Sample Control Bus Creator/3
  Sample Control Bus Creator/1 -> ctrl_out/1
  valid_in/1 -> Delay1/1, Detect Fall Nonpositive/1, Delay/1
  Detect Fall Nonpositive/1 -> Sample Control Bus Creator/2

== system rx2/process divide/transport_block7/Subsystem5/ctrl_gen ==
  data_in : Inport
  valid_in : Inport  Port=2
  Delay : Delay  DelayLength=1  InitialCondition=0
  Delay1 : Delay  DelayLength=1  InitialCondition=0
  Delay2 : Delay  DelayLength=1  InitialCondition=0
  Detect Fall Nonpositive : hdlsllib/Logic and Bit Operations/Detect Fall Nonpositive  vinit=0  OutDataTypeStr=boolean
  Detect Rise Positive : hdlsllib/Logic and Bit Operations/Detect Rise Positive  vinit=0  OutDataTypeStr=boolean
  Sample Control Bus Creator : whdlutilities/Sample Control Bus Creator
  data_out : Outport
  ctrl_out : Outport  Port=2
  wires:
  Detect Rise Positive/1 -> Sample Control Bus Creator/1
  Delay2/1 -> data_out/1
  data_in/1 -> Delay2/1
  Delay1/1 -> Detect Rise Positive/1
  Delay/1 -> Sample Control Bus Creator/3
  Sample Control Bus Creator/1 -> ctrl_out/1
  valid_in/1 -> Delay1/1, Detect Fall Nonpositive/1, Delay/1
  Detect Fall Nonpositive/1 -> Sample Control Bus Creator/2

== system rx2/process divide/transport_block7/Subsystem6/ctrl_gen ==
  data_in : Inport
  valid_in : Inport  Port=2
  Delay : Delay  DelayLength=1  InitialCondition=0
  Delay1 : Delay  DelayLength=1  InitialCondition=0
  Delay2 : Delay  DelayLength=1  InitialCondition=0
  Detect Fall Nonpositive : hdlsllib/Logic and Bit Operations/Detect Fall Nonpositive  vinit=0  OutDataTypeStr=boolean
  Detect Rise Positive : hdlsllib/Logic and Bit Operations/Detect Rise Positive  vinit=0  OutDataTypeStr=boolean
  Sample Control Bus Creator : whdlutilities/Sample Control Bus Creator
  data_out : Outport
  ctrl_out : Outport  Port=2
  wires:
  Detect Rise Positive/1 -> Sample Control Bus Creator/1
  Delay2/1 -> data_out/1
  data_in/1 -> Delay2/1
  Delay1/1 -> Detect Rise Positive/1
  Delay/1 -> Sample Control Bus Creator/3
  Sample Control Bus Creator/1 -> ctrl_out/1
  valid_in/1 -> Delay1/1, Detect Fall Nonpositive/1, Delay/1
  Detect Fall Nonpositive/1 -> Sample Control Bus Creator/2

== system rx2/process divide/transport_block7/Subsystem7/ctrl_gen ==
  data_in : Inport
  valid_in : Inport  Port=2
  Delay : Delay  DelayLength=1  InitialCondition=0
  Delay1 : Delay  DelayLength=1  InitialCondition=0
  Delay2 : Delay  DelayLength=1  InitialCondition=0
  Detect Fall Nonpositive : hdlsllib/Logic and Bit Operations/Detect Fall Nonpositive  vinit=0  OutDataTypeStr=boolean
  Detect Rise Positive : hdlsllib/Logic and Bit Operations/Detect Rise Positive  vinit=0  OutDataTypeStr=boolean
  Sample Control Bus Creator : whdlutilities/Sample Control Bus Creator
  data_out : Outport
  ctrl_out : Outport  Port=2
  wires:
  Detect Rise Positive/1 -> Sample Control Bus Creator/1
  Delay2/1 -> data_out/1
  data_in/1 -> Delay2/1
  Delay1/1 -> Detect Rise Positive/1
  Delay/1 -> Sample Control Bus Creator/3
  Sample Control Bus Creator/1 -> ctrl_out/1
  valid_in/1 -> Delay1/1, Detect Fall Nonpositive/1, Delay/1
  Detect Fall Nonpositive/1 -> Sample Control Bus Creator/2

== system rx2/process divide/transport_block7/Subsystem8/ctrl_gen ==
  data_in : Inport
  valid_in : Inport  Port=2
  Delay : Delay  DelayLength=1  InitialCondition=0
  Delay1 : Delay  DelayLength=1  InitialCondition=0
  Delay2 : Delay  DelayLength=1  InitialCondition=0
  Detect Fall Nonpositive : hdlsllib/Logic and Bit Operations/Detect Fall Nonpositive  vinit=0  OutDataTypeStr=boolean
  Detect Rise Positive : hdlsllib/Logic and Bit Operations/Detect Rise Positive  vinit=0  OutDataTypeStr=boolean
  Sample Control Bus Creator : whdlutilities/Sample Control Bus Creator
  data_out : Outport
  ctrl_out : Outport  Port=2
  wires:
  Detect Rise Positive/1 -> Sample Control Bus Creator/1
  Delay2/1 -> data_out/1
  data_in/1 -> Delay2/1
  Delay1/1 -> Detect Rise Positive/1
  Delay/1 -> Sample Control Bus Creator/3
  Sample Control Bus Creator/1 -> ctrl_out/1
  valid_in/1 -> Delay1/1, Detect Fall Nonpositive/1, Delay/1
  Detect Fall Nonpositive/1 -> Sample Control Bus Creator/2

== system rx2/process divide/transport_block7/Subsystem9/ctrl_gen ==
  data_in : Inport
  valid_in : Inport  Port=2
  Delay : Delay  DelayLength=1  InitialCondition=0
  Delay1 : Delay  DelayLength=1  InitialCondition=0
  Delay2 : Delay  DelayLength=1  InitialCondition=0
  Detect Fall Nonpositive : hdlsllib/Logic and Bit Operations/Detect Fall Nonpositive  vinit=0  OutDataTypeStr=boolean
  Detect Rise Positive : hdlsllib/Logic and Bit Operations/Detect Rise Positive  vinit=0  OutDataTypeStr=boolean
  Sample Control Bus Creator : whdlutilities/Sample Control Bus Creator
  data_out : Outport
  ctrl_out : Outport  Port=2
  wires:
  Detect Rise Positive/1 -> Sample Control Bus Creator/1
  Delay2/1 -> data_out/1
  data_in/1 -> Delay2/1
  Delay1/1 -> Detect Rise Positive/1
  Delay/1 -> Sample Control Bus Creator/3
  Sample Control Bus Creator/1 -> ctrl_out/1
  valid_in/1 -> Delay1/1, Detect Fall Nonpositive/1, Delay/1
  Detect Fall Nonpositive/1 -> Sample Control Bus Creator/2

== system rx2/process divide/transport_block8/Subsystem1/ctrl_gen ==
  data_in : Inport
  valid_in : Inport  Port=2
  Delay : Delay  DelayLength=1  InitialCondition=0
  Delay1 : Delay  DelayLength=1  InitialCondition=0
  Delay2 : Delay  DelayLength=1  InitialCondition=0
  Detect Fall Nonpositive : hdlsllib/Logic and Bit Operations/Detect Fall Nonpositive  vinit=0  OutDataTypeStr=boolean
  Detect Rise Positive : hdlsllib/Logic and Bit Operations/Detect Rise Positive  vinit=0  OutDataTypeStr=boolean
  Sample Control Bus Creator : whdlutilities/Sample Control Bus Creator
  data_out : Outport
  ctrl_out : Outport  Port=2
  wires:
  Detect Rise Positive/1 -> Sample Control Bus Creator/1
  Delay2/1 -> data_out/1
  data_in/1 -> Delay2/1
  Delay1/1 -> Detect Rise Positive/1
  Delay/1 -> Sample Control Bus Creator/3
  Sample Control Bus Creator/1 -> ctrl_out/1
  valid_in/1 -> Delay1/1, Detect Fall Nonpositive/1, Delay/1
  Detect Fall Nonpositive/1 -> Sample Control Bus Creator/2

== system rx2/process divide/transport_block8/Subsystem10/ctrl_gen ==
  data_in : Inport
  valid_in : Inport  Port=2
  Delay : Delay  DelayLength=1  InitialCondition=0
  Delay1 : Delay  DelayLength=1  InitialCondition=0
  Delay2 : Delay  DelayLength=1  InitialCondition=0
  Detect Fall Nonpositive : hdlsllib/Logic and Bit Operations/Detect Fall Nonpositive  vinit=0  OutDataTypeStr=boolean
  Detect Rise Positive : hdlsllib/Logic and Bit Operations/Detect Rise Positive  vinit=0  OutDataTypeStr=boolean
  Sample Control Bus Creator : whdlutilities/Sample Control Bus Creator
  data_out : Outport
  ctrl_out : Outport  Port=2
  wires:
  Detect Fall Nonpositive/1 -> Sample Control Bus Creator/2
  valid_in/1 -> Delay/1, Detect Fall Nonpositive/1, Delay1/1
  Sample Control Bus Creator/1 -> ctrl_out/1
  Delay/1 -> Sample Control Bus Creator/3
  Delay1/1 -> Detect Rise Positive/1
  data_in/1 -> Delay2/1
  Delay2/1 -> data_out/1
  Detect Rise Positive/1 -> Sample Control Bus Creator/1

== system rx2/process divide/transport_block8/Subsystem11/ctrl_gen ==
  data_in : Inport
  valid_in : Inport  Port=2
  Delay : Delay  DelayLength=1  InitialCondition=0
  Delay1 : Delay  DelayLength=1  InitialCondition=0
  Delay2 : Delay  DelayLength=1  InitialCondition=0
  Detect Fall Nonpositive : hdlsllib/Logic and Bit Operations/Detect Fall Nonpositive  vinit=0  OutDataTypeStr=boolean
  Detect Rise Positive : hdlsllib/Logic and Bit Operations/Detect Rise Positive  vinit=0  OutDataTypeStr=boolean
  Sample Control Bus Creator : whdlutilities/Sample Control Bus Creator
  data_out : Outport
  ctrl_out : Outport  Port=2
  wires:
  Detect Fall Nonpositive/1 -> Sample Control Bus Creator/2
  valid_in/1 -> Delay/1, Detect Fall Nonpositive/1, Delay1/1
  Sample Control Bus Creator/1 -> ctrl_out/1
  Delay/1 -> Sample Control Bus Creator/3
  Delay1/1 -> Detect Rise Positive/1
  data_in/1 -> Delay2/1
  Delay2/1 -> data_out/1
  Detect Rise Positive/1 -> Sample Control Bus Creator/1

== system rx2/process divide/transport_block8/Subsystem12/ctrl_gen ==
  data_in : Inport
  valid_in : Inport  Port=2
  Delay : Delay  DelayLength=1  InitialCondition=0
  Delay1 : Delay  DelayLength=1  InitialCondition=0
  Delay2 : Delay  DelayLength=1  InitialCondition=0
  Detect Fall Nonpositive : hdlsllib/Logic and Bit Operations/Detect Fall Nonpositive  vinit=0  OutDataTypeStr=boolean
  Detect Rise Positive : hdlsllib/Logic and Bit Operations/Detect Rise Positive  vinit=0  OutDataTypeStr=boolean
  Sample Control Bus Creator : whdlutilities/Sample Control Bus Creator
  data_out : Outport
  ctrl_out : Outport  Port=2
  wires:
  Detect Fall Nonpositive/1 -> Sample Control Bus Creator/2
  valid_in/1 -> Delay/1, Detect Fall Nonpositive/1, Delay1/1
  Sample Control Bus Creator/1 -> ctrl_out/1
  Delay/1 -> Sample Control Bus Creator/3
  Delay1/1 -> Detect Rise Positive/1
  data_in/1 -> Delay2/1
  Delay2/1 -> data_out/1
  Detect Rise Positive/1 -> Sample Control Bus Creator/1

== system rx2/process divide/transport_block8/Subsystem13/ctrl_gen ==
  data_in : Inport
  valid_in : Inport  Port=2
  Delay : Delay  DelayLength=1  InitialCondition=0
  Delay1 : Delay  DelayLength=1  InitialCondition=0
  Delay2 : Delay  DelayLength=1  InitialCondition=0
  Detect Fall Nonpositive : hdlsllib/Logic and Bit Operations/Detect Fall Nonpositive  vinit=0  OutDataTypeStr=boolean
  Detect Rise Positive : hdlsllib/Logic and Bit Operations/Detect Rise Positive  vinit=0  OutDataTypeStr=boolean
  Sample Control Bus Creator : whdlutilities/Sample Control Bus Creator
  data_out : Outport
  ctrl_out : Outport  Port=2
  wires:
  Detect Fall Nonpositive/1 -> Sample Control Bus Creator/2
  valid_in/1 -> Delay/1, Detect Fall Nonpositive/1, Delay1/1
  Sample Control Bus Creator/1 -> ctrl_out/1
  Delay/1 -> Sample Control Bus Creator/3
  Delay1/1 -> Detect Rise Positive/1
  data_in/1 -> Delay2/1
  Delay2/1 -> data_out/1
  Detect Rise Positive/1 -> Sample Control Bus Creator/1

== system rx2/process divide/transport_block8/Subsystem14/ctrl_gen ==
  data_in : Inport
  valid_in : Inport  Port=2
  Delay : Delay  DelayLength=1  InitialCondition=0
  Delay1 : Delay  DelayLength=1  InitialCondition=0
  Delay2 : Delay  DelayLength=1  InitialCondition=0
  Detect Fall Nonpositive : hdlsllib/Logic and Bit Operations/Detect Fall Nonpositive  vinit=0  OutDataTypeStr=boolean
  Detect Rise Positive : hdlsllib/Logic and Bit Operations/Detect Rise Positive  vinit=0  OutDataTypeStr=boolean
  Sample Control Bus Creator : whdlutilities/Sample Control Bus Creator
  data_out : Outport
  ctrl_out : Outport  Port=2
  wires:
  Detect Fall Nonpositive/1 -> Sample Control Bus Creator/2
  valid_in/1 -> Delay/1, Detect Fall Nonpositive/1, Delay1/1
  Sample Control Bus Creator/1 -> ctrl_out/1
  Delay/1 -> Sample Control Bus Creator/3
  Delay1/1 -> Detect Rise Positive/1
  data_in/1 -> Delay2/1
  Delay2/1 -> data_out/1
  Detect Rise Positive/1 -> Sample Control Bus Creator/1

== system rx2/process divide/transport_block8/Subsystem2/ctrl_gen ==
  data_in : Inport
  valid_in : Inport  Port=2
  Delay : Delay  DelayLength=1  InitialCondition=0
  Delay1 : Delay  DelayLength=1  InitialCondition=0
  Delay2 : Delay  DelayLength=1  InitialCondition=0
  Detect Fall Nonpositive : hdlsllib/Logic and Bit Operations/Detect Fall Nonpositive  vinit=0  OutDataTypeStr=boolean
  Detect Rise Positive : hdlsllib/Logic and Bit Operations/Detect Rise Positive  vinit=0  OutDataTypeStr=boolean
  Sample Control Bus Creator : whdlutilities/Sample Control Bus Creator
  data_out : Outport
  ctrl_out : Outport  Port=2
  wires:
  Detect Fall Nonpositive/1 -> Sample Control Bus Creator/2
  valid_in/1 -> Delay/1, Detect Fall Nonpositive/1, Delay1/1
  Sample Control Bus Creator/1 -> ctrl_out/1
  Delay/1 -> Sample Control Bus Creator/3
  Delay1/1 -> Detect Rise Positive/1
  data_in/1 -> Delay2/1
  Delay2/1 -> data_out/1
  Detect Rise Positive/1 -> Sample Control Bus Creator/1

== system rx2/process divide/transport_block8/Subsystem3/ctrl_gen ==
  data_in : Inport
  valid_in : Inport  Port=2
  Delay : Delay  DelayLength=1  InitialCondition=0
  Delay1 : Delay  DelayLength=1  InitialCondition=0
  Delay2 : Delay  DelayLength=1  InitialCondition=0
  Detect Fall Nonpositive : hdlsllib/Logic and Bit Operations/Detect Fall Nonpositive  vinit=0  OutDataTypeStr=boolean
  Detect Rise Positive : hdlsllib/Logic and Bit Operations/Detect Rise Positive  vinit=0  OutDataTypeStr=boolean
  Sample Control Bus Creator : whdlutilities/Sample Control Bus Creator
  data_out : Outport
  ctrl_out : Outport  Port=2
  wires:
  Detect Rise Positive/1 -> Sample Control Bus Creator/1
  Delay2/1 -> data_out/1
  data_in/1 -> Delay2/1
  Delay1/1 -> Detect Rise Positive/1
  Delay/1 -> Sample Control Bus Creator/3
  Sample Control Bus Creator/1 -> ctrl_out/1
  valid_in/1 -> Delay1/1, Detect Fall Nonpositive/1, Delay/1
  Detect Fall Nonpositive/1 -> Sample Control Bus Creator/2
